simulink model "backup_test1"  (R2016a)
settings: Solver=ode4  StartTime=0.0  StopTime=inf  RelTol=1e-3
libraries: xpcmeasurementcomputinglib x7, slrtlib x6, xpcconteclib x2, xpcutilitieslib x1, xpcrtudplib x1
settings Model: SimulationMode=external  Creator=Biorobotics  LastModifiedBy=Biorobotics
settings SolverCC: EnableConcurrentExecution=on
settings DataIOCC: SaveFormat=StructureWithTime
settings OptimizationCC: BlockReduction=off  OptimizeBlockIOStorage=off  BufferReuse=off  GlobalBufferReuse=off  ExpressionFolding=off  LocalBlockOutputs=off
settings HardwareCC: ProdBitPerPointer=32  ProdLargestAtomicFloat=None  ProdWordSize=32  ProdLongLongMode=on  ProdHWDeviceType=Generic->32-bit x86 compatible
settings RTWCC: SystemTargetFile=slrt.tlc  TemplateMakefile=slrt_default_tmf  Description=Simulink Real-Time  RTWCompilerOptimization=on

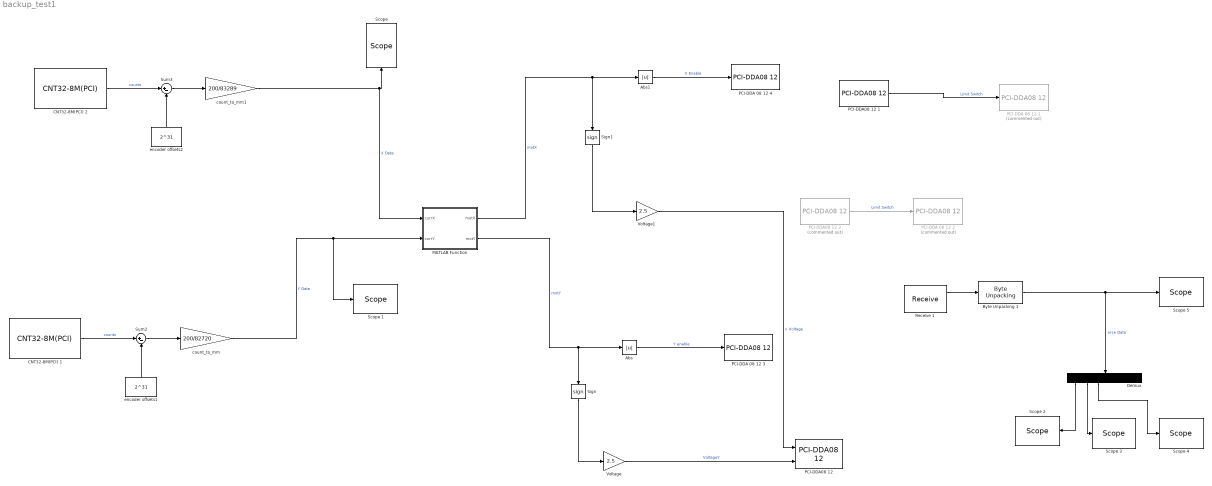
== system backup_test1 ==
  Abs : Abs
  Abs1 : Abs
  Byte Unpacking 1 : xpcutilitieslib/Byte Unpacking   MaskUnpackedDataTypes={'double'}  MaskUnpackedDataSizes={[6]}  MaskAlignment=1
  CNT32-8M(PCI) 1 : xpcconteclib/Incremental Encoder/CNT32-8M(PCI)   Channel=2  OperationMode=2-phase Input Synchronous Clear Multiply by 4  DigitalFilter=No filtering  PulseInput=TTL level input  Direction=Up in the clockwise direction/Down in the counterclockwise direction  InitialValue=2^31  LoadInitialValue=on  SampleTime=0.001  PciSlot=[4 5]  StartMethod=Model Start  StopMethod=Model Terminate  ZeroClearRising=off  ZeroClearFalling=off  ZeroClearMatch0=off  ZeroClearMatch1=off  PresetRising=off  PresetFalling=off  PresetMatch0=off  PresetMatch1=off  PresetValue=0  Match0Value=0  Match1Value=0  OutputSignalMatch0=off  OutputSignalMatch1=off  OutputSignalAbnormal=off  OutputSignalDigitalFilter=off  OutputSignalAlarm=off  OneShotDuration=10 microseconds  IndexEnable=Disable  IndexLogic=Positive (Active High)  EnableDigitalInput=off  EnableDigitalOutput=off  DigitalOutputInitialValue=None  DigitalOutputFinalValue=None
  CNT32-8M(PCI) 2 : xpcconteclib/Incremental Encoder/CNT32-8M(PCI)   Channel=1  OperationMode=2-phase Input Synchronous Clear Multiply by 4  DigitalFilter=No filtering  PulseInput=TTL level input  Direction=Up in the clockwise direction/Down in the counterclockwise direction  InitialValue=2^31  LoadInitialValue=on  SampleTime=0.001  PciSlot=[4 5]  StartMethod=Model Start  StopMethod=Model Terminate  ZeroClearRising=off  ZeroClearFalling=off  ZeroClearMatch0=off  ZeroClearMatch1=off  PresetRising=off  PresetFalling=off  PresetMatch0=off  PresetMatch1=off  PresetValue=0  Match0Value=0  Match1Value=0  OutputSignalMatch0=off  OutputSignalMatch1=off  OutputSignalAbnormal=off  OutputSignalDigitalFilter=off  OutputSignalAlarm=off  OneShotDuration=10 microseconds  IndexEnable=Disable  IndexLogic=Positive (Active High)  EnableDigitalInput=off  EnableDigitalOutput=off  DigitalOutputInitialValue=None  DigitalOutputFinalValue=None
  Demux : Demux  Outputs=6
  MATLAB Function : MATLAB Function  TreatAsAtomicUnit=on
  PCI-DDA 08 12 1 : xpcmeasurementcomputinglib/Digital Output/PCI-DDA08 12   Commented=on  channel=1  port=A  reset=[1]  initValue=[0]  chip=1  sampletime=0.001  slot=-1
  PCI-DDA 08 12 2 : xpcmeasurementcomputinglib/Digital Output/PCI-DDA08 12   Commented=on  channel=3  port=A  reset=[1]  initValue=[0]  chip=1  sampletime=0.001  slot=-1
  PCI-DDA 08 12 3 : xpcmeasurementcomputinglib/Digital Output/PCI-DDA08 12   channel=3  port=A  reset=[1]  initValue=[0]  chip=1  sampletime=0.001  slot=-1
  PCI-DDA 08 12 4 : xpcmeasurementcomputinglib/Digital Output/PCI-DDA08 12   channel=1  port=A  reset=[1]  initValue=[0]  chip=1  sampletime=0.001  slot=-1
  "PCI-DDA08 12 " : xpcmeasurementcomputinglib/D//A/PCI-DDA08 12   channel=[1 2]  range=[-10 -10]  reset=[1]  initValue=[0]  sampletime=0.001  pci_dev=-1
  PCI-DDA08 12 1 : xpcmeasurementcomputinglib/Digital Input/PCI-DDA08 12   channel=6  port=A  chip=2  sampletime=0.001  slot=-1
  PCI-DDA08 12 3 : xpcmeasurementcomputinglib/Digital Input/PCI-DDA08 12   Commented=on  channel=6  port=B  chip=2  sampletime=0.001  slot=-1
  Receive 1 : xpcrtudplib/Legacy UDP/Receive   ipAddress=192.168.1.2  ipPort=25000  width=48  vblLen=off  sampletime=0.001
  "Scope " : slrtlib/Displays and Logging/Scope   scopeno=1  scopetype=File  autostart=on  viewmode=Graphical redraw  formatstr='%15.6f'  grid=on  ylimits=[0,0]  nosamples=200000  noprepostsamples=0  interleave=1  triggermode=FreeRun  triggersignal=1  trigsignalfromport=off  triggerlevel=0.0  triggerslope=Either  triggerscope=1  triggersample=0  filename=Xdata.dat  mode=Lazy  writesize=512  autorestart=off  dynamicfilemode=off  maxwritefilesize=512*1024^2
  Scope 1 : slrtlib/Displays and Logging/Scope   scopeno=2  scopetype=File  autostart=on  viewmode=Graphical redraw  formatstr='%15.6f'  grid=on  ylimits=[0,0]  nosamples=200000  noprepostsamples=0  interleave=1  triggermode=FreeRun  triggersignal=1  trigsignalfromport=off  triggerlevel=0.0  triggerslope=Either  triggerscope=1  triggersample=0  filename=Ydata.dat  mode=Lazy  writesize=512  autorestart=off  dynamicfilemode=off  maxwritefilesize=512*1024^2
  Scope 2 : slrtlib/Displays and Logging/Scope   scopeno=3  scopetype=File  autostart=on  viewmode=Graphical redraw  formatstr='%15.6f'  grid=on  ylimits=[0,0]  nosamples=200000  noprepostsamples=0  interleave=1  triggermode=FreeRun  triggersignal=1  trigsignalfromport=off  triggerlevel=0.0  triggerslope=Either  triggerscope=1  triggersample=0  filename=FXdata.dat  mode=Lazy  writesize=512  autorestart=off  dynamicfilemode=off  maxwritefilesize=512*1024^2
  Scope 3 : slrtlib/Displays and Logging/Scope   scopeno=4  scopetype=File  autostart=on  viewmode=Graphical redraw  formatstr='%15.6f'  grid=on  ylimits=[0,0]  nosamples=200000  noprepostsamples=0  interleave=1  triggermode=FreeRun  triggersignal=1  trigsignalfromport=off  triggerlevel=0.0  triggerslope=Either  triggerscope=1  triggersample=0  filename=Fydata.dat  mode=Lazy  writesize=512  autorestart=off  dynamicfilemode=off  maxwritefilesize=512*1024^2
  Scope 4 : slrtlib/Displays and Logging/Scope   scopeno=5  scopetype=File  autostart=on  viewmode=Graphical redraw  formatstr='%15.6f'  grid=on  ylimits=[0,0]  nosamples=200000  noprepostsamples=0  interleave=1  triggermode=FreeRun  triggersignal=1  trigsignalfromport=off  triggerlevel=0.0  triggerslope=Either  triggerscope=1  triggersample=0  filename=Fzdata.dat  mode=Lazy  writesize=512  autorestart=off  dynamicfilemode=off  maxwritefilesize=512*1024^2
  Scope 5 : slrtlib/Displays and Logging/Scope   scopeno=6  scopetype=Target  autostart=on  viewmode=Graphical rolling  formatstr='%15.6f'  grid=on  ylimits=[0,0]  nosamples=10000  noprepostsamples=0  interleave=1  triggermode=FreeRun  triggersignal=1  trigsignalfromport=off  triggerlevel=0.0  triggerslope=Either  triggerscope=1  triggersample=0  filename=Fzdata1.dat  mode=Lazy  writesize=512  autorestart=off  dynamicfilemode=off  maxwritefilesize=512*1024^2
  Sign : Signum
  Sign1 : Signum
  Sum2 : Sum  Inputs=|+-
  Sum3 : Sum  Inputs=|+-
  Voltage : Gain  Gain=2.5
  Voltage1 : Gain  Gain=2.5
  count_to_mm : Gain  Gain=200/82720
  count_to_mm1 : Gain  Gain=200/83289
  encoder offsets1 : Constant  Value=2^31
  encoder offsets2 : Constant  Value=2^31
  wires:
  PCI-DDA08 12 1/1 -> PCI-DDA 08 12 1/1  "Limit Switch"
  Voltage/1 -> "PCI-DDA08 12 "/2  "VoltageY"
  encoder offsets1/1 -> Sum2/2
  CNT32-8M(PCI) 1/1 -> Sum2/1  "counts"
  Sum2/1 -> count_to_mm/1
  PCI-DDA08 12 3/1 -> PCI-DDA 08 12 2/1  "Limit Switch"
  Abs/1 -> PCI-DDA 08 12 3/1  "Y enable"
  Sign/1 -> Voltage/1
  Voltage1/1 -> "PCI-DDA08 12 "/1  "x Voltage"
  encoder offsets2/1 -> Sum3/2
  CNT32-8M(PCI) 2/1 -> Sum3/1  "counts"
  Sum3/1 -> count_to_mm1/1
  Abs1/1 -> PCI-DDA 08 12 4/1  "X Enable"
  Sign1/1 -> Voltage1/1
  MATLAB Function/1(motX) -> Sign1/1, Abs1/1  "motX"
  MATLAB Function/2(motY) -> Sign/1, Abs/1  "motY"
  Receive 1/1 -> Byte Unpacking 1/1
  Byte Unpacking 1/1 -> Scope 5/1, Demux/1  "orce Data"
  count_to_mm/1 -> Scope 1/1, MATLAB Function/2(currY)  "Y Data"
  count_to_mm1/1 -> MATLAB Function/1(currX), "Scope "/1  "X Data"
  Demux/1 -> Scope 2/1
  Demux/2 -> Scope 3/1
  Demux/3 -> Scope 4/1

== matlab function backup_test1/MATLAB Function ==
  data: currX input; motX output; currY input; motY output
function [motX,motY] = moveRas(currX,currY)
%#codegen
%#codegen
currX = ceil(currX);
currY = ceil(currY);
nIntervals=2;
remY = mod(currY,nIntervals);
quotY = currY/nIntervals;
motX = 0;
motY = 0;
maxX = 87;
minX = 0;
maxY=87;

if(currX>maxX)
    maxX = currX;
end
if(currX<minX)
    minX = currX;
end

if((currX>=minX)&&(currX<maxX)&&(remY==0)&&(mod(quotY,2)==0))
    motX = -1;
elseif((currX>minX)&&(currX<=maxX)&&(remY==0)&&(mod(quotY,2)==1))
    motX = 1;
elseif(((currX==minX)||(currX>=maxX))&&(remY~=0))
    motY = -1;
elseif((currX==minX)&&(remY==0)&&(mod(quotY,2)==1))
    motY = -1;
elseif((currX>=maxX)&&(remY==0)&&(mod(quotY,2)==0))
    motY=-1;
end

if((currY>maxY))
    motX = 0;
    motY = 0;
end

end
